simulink model "simulation"  (R2020b)
settings: Solver=VariableStepAuto  StartTime=0.0  StopTime=10  RelTol=1e-3
values from neighbouring files (symbols this model uses):
  delta = geometry(y, x, dx, delta0)    [main.m]
  dx = (x_min:0.0001:x_max)    [main.m]
  Q = actuator_load(rho, S, delta, v)    [main.m]
  v = linspace(v_min, v_max, 100)    [main.m]
settings Model: Creator=HP  LastModifiedBy=HP

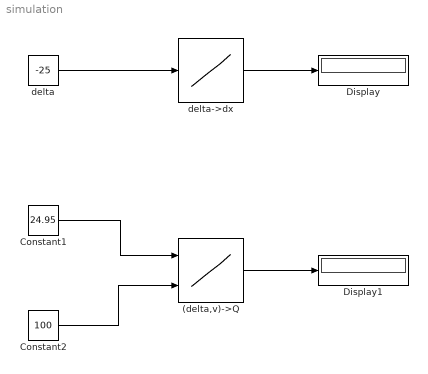
== system simulation ==
  (delta,v)->Q : Lookup_n-D  BreakpointsForDimension1=delta  BreakpointsForDimension2=v  BreakpointsForDimension1FirstPoint=0.007949390000000002  Table=Q  InternalRulePriority=Speed  RndMeth=Simplest  InputSameDT=on
      settings: InputPortMap=u0,u1
  Constant1 : Constant  Value=24.95
  Constant2 : Constant  Value=100
  Display : Display
  Display1 : Display
  delta : Constant  Value=-25
  delta->dx : Lookup_n-D  NumberOfTableDimensions=1  BreakpointsForDimension1=delta  BreakpointsForDimension1FirstPoint=0.007949390000000002  Table=dx  InternalRulePriority=Speed  RndMeth=Simplest  InputSameDT=on
  wires:
  delta->dx/1 -> Display/1
  delta/1 -> delta->dx/1
  Constant1/1 -> (delta,v)->Q/1
  Constant2/1 -> (delta,v)->Q/2
  (delta,v)->Q/1 -> Display1/1
